simulink model "gm_dvfs_zed_simple"  (R2025b)
settings: Solver=FixedStepDiscrete  StartTime=0.0  StopTime=10.0  FixedStep=0.1  RelTol=1e-3
libraries: simulink x3
settings Model: Creator=Vimal Rency  LastModifiedBy=Vimal Rency
settings OptimizationCC: BlockReduction=off  ConditionallyExecuteInputs=off  DefaultParameterBehavior=Inlined
settings DebuggingCC: InheritedTsInSrcMsg=none
settings HardwareCC: ProdBitPerPointer=32.0  ProdBitPerSizeT=32.0  ProdBitPerPtrDiffT=32.0  ProdLargestAtomicFloat=None  ProdIntDivRoundTo=Undefined  ProdEndianess=Unspecified  ProdWordSize=32.0  ProdHWDeviceType=ASIC/FPGA->ASIC/FPGA  TargetBitPerPointer=64.0  TargetBitPerSizeT=64.0  TargetBitPerPtrDiffT=64.0  TargetLongLongMode=on  TargetIntDivRoundTo=Zero  TargetEndianess=LittleEndian  TargetWordSize=64.0  TargetHWDeviceType=Custom Processor->MATLAB Host Computer  ProdEqTarget=off

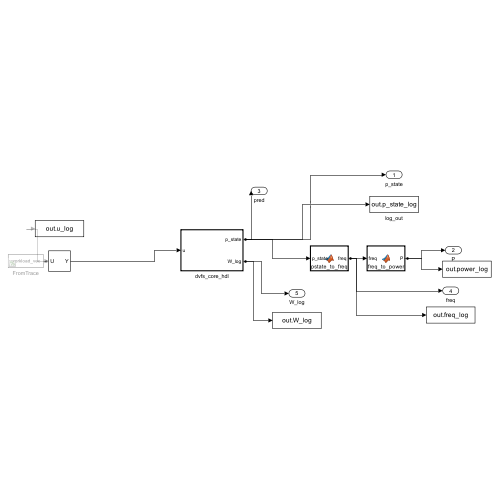
[thumbnail: Simulink's stored preview of the top-level diagram]
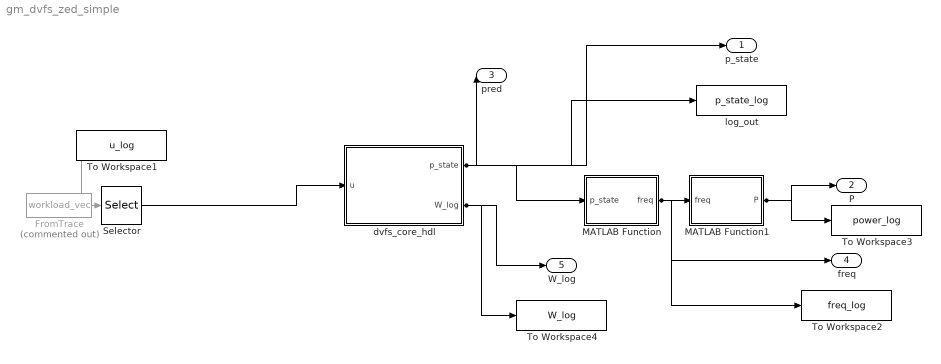
== system gm_dvfs_zed_simple ==
  FromTrace : FromWorkspace  Commented=on  VariableName=workload_vec
  MATLAB Function : MATLAB Function  TreatAsAtomicUnit=on
  MATLAB Function1 : MATLAB Function  TreatAsAtomicUnit=on
  Selector : Selector  NumberOfDimensions=2  InputPortWidth=3  IndexOptions=Select all,Index vector (dialog)  Indices=[1 3],1  OutputSizes=1,1
  To Workspace1 : ToWorkspace  VariableName=u_log  SampleTime=-1
  To Workspace2 : ToWorkspace  VariableName=freq_log  SampleTime=-1
  To Workspace3 : ToWorkspace  VariableName=power_log  SampleTime=-1
  To Workspace4 : ToWorkspace  VariableName=W_log  SampleTime=-1
  dvfs_core_hdl : Subsystem  TreatAsAtomicUnit=on
  log_out : ToWorkspace  VariableName=p_state_log  SampleTime=-1
  p_state : Outport
  P : Outport  Port=2
  pred : Outport  Port=3
  freq : Outport  Port=4
  W_log : Outport  Port=5
  wires:
  Selector/1 -> dvfs_core_hdl/1(u)
  dvfs_core_hdl/1(p_state) -> log_out/1, p_state/1, MATLAB Function/1(p_state), pred/1
  dvfs_core_hdl/2(W_log) -> W_log/1, To Workspace4/1
  MATLAB Function/1(freq) -> MATLAB Function1/1(freq), To Workspace2/1, freq/1
  MATLAB Function1/1(P) -> To Workspace3/1, P/1
  FromTrace/1 -> Selector/1, To Workspace1/1

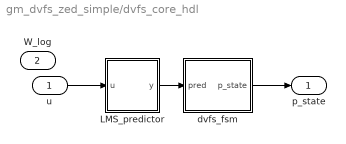
== system gm_dvfs_zed_simple/dvfs_core_hdl ==
  u : Inport  OutDataTypeStr=double  PortDimensions=1  SampleTime=0.1
  LMS_predictor : Subsystem
  dvfs_fsm : Subsystem
  p_state : Outport  SampleTime=0.1
  W_log : Outport  Port=2  SampleTime=0.1
  wires:
  u/1 -> LMS_predictor/1(u)
  LMS_predictor/1(y) -> dvfs_fsm/1(pred)
  dvfs_fsm/1(p_state) -> p_state/1

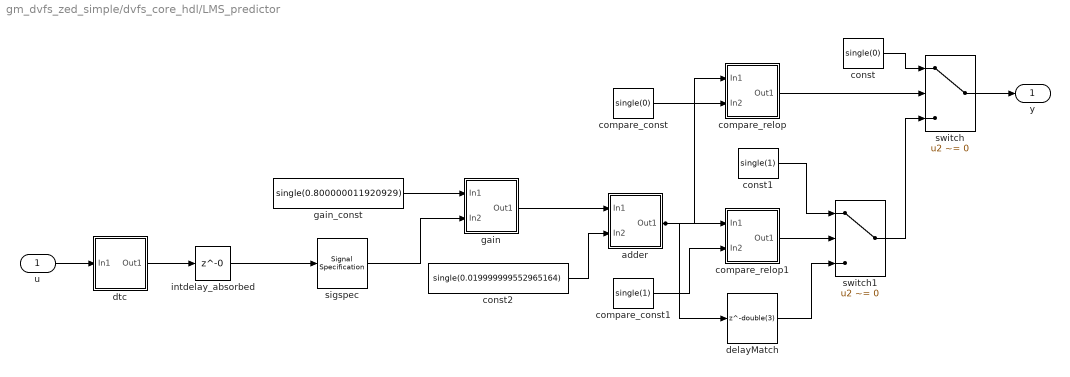
== system gm_dvfs_zed_simple/dvfs_core_hdl/LMS_predictor ==
  u : Inport  OutDataTypeStr=double  PortDimensions=1  SampleTime=0.1
  adder : Subsystem
      mask Display: disp('NFP\nadd');
  compare_const : Constant  Value=single(0)  OutDataTypeStr=single  SampleTime=0.1
  compare_const1 : Constant  Value=single(1)  OutDataTypeStr=single  SampleTime=0.1
  compare_relop : Subsystem
      mask Display: disp('NFP\nrelop');
  compare_relop1 : Subsystem
      mask Display: disp('NFP\nrelop');
  const : Constant  Value=single(0)  VectorParams1D=off  OutDataTypeStr=single  SampleTime=0.1
  const1 : Constant  Value=single(1)  VectorParams1D=off  OutDataTypeStr=single  SampleTime=0.1
  const2 : Constant  Value=single(0.019999999552965164)  VectorParams1D=off  OutDataTypeStr=single  SampleTime=0.1
  delayMatch : Delay  DelayLength=double(3)  InitialCondition=0  SampleTime=0.1
  dtc : Subsystem
      mask Display: disp('NFP\nconv');
  gain : Subsystem
      mask Display: disp('NFP\nmul');
  gain_const : Constant  Value=single(0.800000011920929)  OutDataTypeStr=single  SampleTime=0.1
  intdelay_absorbed : Delay  DelayLength=0
  sigspec : SignalSpecification  OutDataTypeStr=single  Dimensions=1
  switch : Switch  Criteria=u2 ~= 0  Threshold="fi(0,0,1,0,\"hex\",\"0\")"  OutDataTypeStr=single  SampleTime=0.1  SaturateOnIntegerOverflow=off  InputSameDT=off
  switch1 : Switch  Criteria=u2 ~= 0  Threshold="fi(0,0,1,0,\"hex\",\"0\")"  OutDataTypeStr=single  SampleTime=0.1  SaturateOnIntegerOverflow=off  InputSameDT=off
  y : Outport  SampleTime=0.1
  wires:
  u/1 -> dtc/1(In1)
  dtc/1(Out1) -> intdelay_absorbed/1
  intdelay_absorbed/1 -> sigspec/1
  gain_const/1 -> gain/1(In1)
  gain/1(Out1) -> adder/1(In1)
  sigspec/1 -> gain/2(In2)
  const2/1 -> adder/2(In2)
  compare_const/1 -> compare_relop/2(In2)
  adder/1(Out1) -> compare_relop1/1(In1), compare_relop/1(In1), delayMatch/1
  compare_const1/1 -> compare_relop1/2(In2)
  compare_relop/1(Out1) -> switch/2
  const1/1 -> switch1/1
  compare_relop1/1(Out1) -> switch1/2
  delayMatch/1 -> switch1/3
  const/1 -> switch/1
  switch1/1 -> switch/3
  switch/1 -> y/1

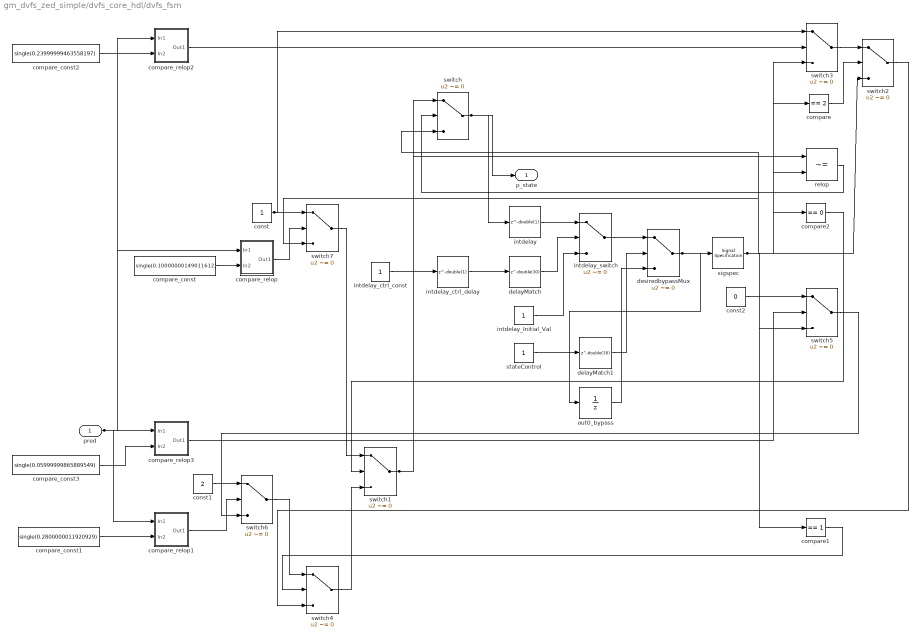
== system gm_dvfs_zed_simple/dvfs_core_hdl/dvfs_fsm ==
  pred : Inport  OutDataTypeStr=single  PortDimensions=1  SampleTime=0.1
  compare : simulink/Logic and Bit Operations/Compare To Constant  relop===  const=2  OutDataTypeStr=boolean
  compare1 : simulink/Logic and Bit Operations/Compare To Constant  relop===  const=1  OutDataTypeStr=boolean
  compare2 : simulink/Logic and Bit Operations/Compare To Constant  relop===  const=0  OutDataTypeStr=boolean
  compare_const : Constant  Value=single(0.10000000149011612)  OutDataTypeStr=single  SampleTime=0.1
  compare_const1 : Constant  Value=single(0.2800000011920929)  OutDataTypeStr=single  SampleTime=0.1
  compare_const2 : Constant  Value=single(0.23999999463558197)  OutDataTypeStr=single  SampleTime=0.1
  compare_const3 : Constant  Value=single(0.05999999865889549)  OutDataTypeStr=single  SampleTime=0.1
  compare_relop : Subsystem
      mask Display: disp('NFP\nrelop');
  compare_relop1 : Subsystem
      mask Display: disp('NFP\nrelop');
  compare_relop2 : Subsystem
      mask Display: disp('NFP\nrelop');
  compare_relop3 : Subsystem
      mask Display: disp('NFP\nrelop');
  const : Constant  VectorParams1D=off  OutDataTypeStr=uint8  SampleTime=0.1
  const1 : Constant  Value=2  VectorParams1D=off  OutDataTypeStr=uint8  SampleTime=0.1
  const2 : Constant  Value=0  VectorParams1D=off  OutDataTypeStr=uint8  SampleTime=0.1
  delayMatch : Delay  DelayLength=double(30)  InitialCondition=0  SampleTime=0.1
  delayMatch1 : Delay  DelayLength=double(30)  InitialCondition=0  SampleTime=0.1
  desiredbypassMux : Switch  Criteria=u2 ~= 0  Threshold=double(0)  OutDataTypeStr=uint8  SampleTime=0.1  SaturateOnIntegerOverflow=off  InputSameDT=off
  intdelay : Delay  DelayLength=double(1)  InitialCondition=0  SampleTime=0.1
  intdelay_Initial_Val : Constant  OutDataTypeStr=uint8  SampleTime=0.1
  intdelay_ctrl_const : Constant  OutDataTypeStr=boolean  SampleTime=0.1
  intdelay_ctrl_delay : Delay  DelayLength=double(1)  InitialCondition=0  SampleTime=0.1
  intdelay_switch : Switch  Criteria=u2 ~= 0  Threshold=double(0)  OutDataTypeStr=uint8  SampleTime=0.1  SaturateOnIntegerOverflow=off  InputSameDT=off
  out0_bypass : UnitDelay  SampleTime=0.1
  relop : RelationalOperator  Operator=~=  OutDataTypeStr=boolean  SampleTime=0.1  InputSameDT=off
  sigspec : SignalSpecification  OutDataTypeStr=uint8  Dimensions=1
  stateControl : Constant  OutDataTypeStr=boolean  SampleTime=0.1
  switch{,1..7} (8 alike) : Switch  Criteria=u2 ~= 0  Threshold="fi(0,0,1,0,\"hex\",\"0\")"  OutDataTypeStr=uint8  SampleTime=0.1  SaturateOnIntegerOverflow=off  InputSameDT=off
  p_state : Outport  SampleTime=0.1
  wires:
  const1/1 -> switch6/1
  switch7/1 -> switch1/1
  compare_const2/1 -> compare_relop2/2(In2)
  pred/1 -> compare_relop3/1(In1), compare_relop2/1(In1), compare_relop1/1(In1), compare_relop/1(In1)
  compare_const1/1 -> compare_relop1/2(In2)
  compare_const3/1 -> compare_relop3/2(In2)
  compare_relop2/1(Out1) -> switch3/2
  compare_const/1 -> compare_relop/2(In2)
  compare_relop3/1(Out1) -> switch5/2
  compare_relop1/1(Out1) -> switch6/2
  switch3/1 -> switch2/1
  const/1 -> switch7/1, switch3/1
  const2/1 -> switch5/1
  compare_relop/1(Out1) -> switch7/2
  switch6/1 -> switch4/1
  switch4/1 -> switch1/3
  switch2/1 -> switch4/3
  intdelay_ctrl_const/1 -> intdelay_ctrl_delay/1
  switch1/1 -> switch/1, relop/1
  switch/1 -> p_state/1, intdelay/1
  intdelay_ctrl_delay/1 -> delayMatch/1
  intdelay/1 -> intdelay_switch/1
  delayMatch/1 -> intdelay_switch/2
  intdelay_Initial_Val/1 -> intdelay_switch/3
  stateControl/1 -> delayMatch1/1
  intdelay_switch/1 -> desiredbypassMux/1
  delayMatch1/1 -> desiredbypassMux/2
  out0_bypass/1 -> desiredbypassMux/3
  desiredbypassMux/1 -> out0_bypass/1, sigspec/1
  sigspec/1 -> switch7/3, switch/3, switch2/3, switch5/3, switch3/3, compare1/1, compare/1, compare2/1, relop/2
  compare/1 -> switch2/2
  relop/1 -> switch/2
  compare2/1 -> switch1/2
  switch5/1 -> switch6/3
  compare1/1 -> switch4/2

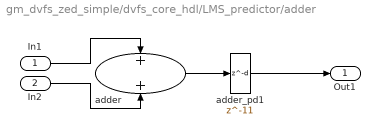
== system gm_dvfs_zed_simple/dvfs_core_hdl/LMS_predictor/adder ==
  In1 : Inport
  In2 : Inport  Port=2
  adder : Sum  OutDataTypeStr=single  SampleTime=0.1
  adder_pd1 : Delay  DelayLength=11
  Out1 : Outport
  wires:
  In1/1 -> adder/1
  In2/1 -> adder/2
  adder/1 -> adder_pd1/1
  adder_pd1/1 -> Out1/1

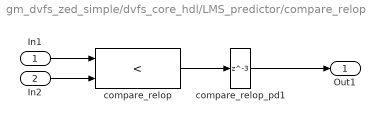
== system gm_dvfs_zed_simple/dvfs_core_hdl/LMS_predictor/compare_relop ==
  In1 : Inport
  In2 : Inport  Port=2
  compare_relop : RelationalOperator  Operator=<  OutDataTypeStr=boolean  SampleTime=0.1
  compare_relop_pd1 : Delay  DelayLength=3
  Out1 : Outport
  wires:
  In1/1 -> compare_relop/1
  In2/1 -> compare_relop/2
  compare_relop/1 -> compare_relop_pd1/1
  compare_relop_pd1/1 -> Out1/1

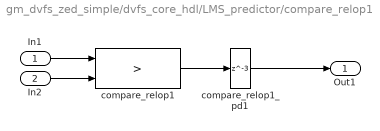
== system gm_dvfs_zed_simple/dvfs_core_hdl/LMS_predictor/compare_relop1 ==
  In1 : Inport
  In2 : Inport  Port=2
  compare_relop1 : RelationalOperator  Operator=>  OutDataTypeStr=boolean  SampleTime=0.1
  compare_relop1_pd1 : Delay  DelayLength=3
  Out1 : Outport
  wires:
  In1/1 -> compare_relop1/1
  In2/1 -> compare_relop1/2
  compare_relop1/1 -> compare_relop1_pd1/1
  compare_relop1_pd1/1 -> Out1/1

== system gm_dvfs_zed_simple/dvfs_core_hdl/LMS_predictor/dtc ==
  In1 : Inport
  dtc : DataTypeConversion  OutDataTypeStr=single  SampleTime=0.1  SaturateOnIntegerOverflow=off  RndMeth=Floor
  dtc_pd1 : Delay  DelayLength=6
  Out1 : Outport
  wires:
  In1/1 -> dtc/1
  dtc/1 -> dtc_pd1/1
  dtc_pd1/1 -> Out1/1

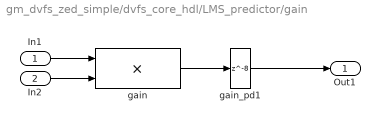
== system gm_dvfs_zed_simple/dvfs_core_hdl/LMS_predictor/gain ==
  In1 : Inport
  In2 : Inport  Port=2
  gain : Product  Inputs=**  OutDataTypeStr=single  SampleTime=0.1
  gain_pd1 : Delay  DelayLength=8
  Out1 : Outport
  wires:
  In1/1 -> gain/1
  In2/1 -> gain/2
  gain/1 -> gain_pd1/1
  gain_pd1/1 -> Out1/1

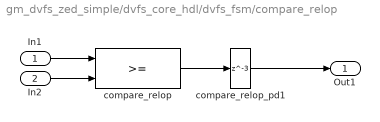
== system gm_dvfs_zed_simple/dvfs_core_hdl/dvfs_fsm/compare_relop ==
  In1 : Inport
  In2 : Inport  Port=2
  compare_relop : RelationalOperator  OutDataTypeStr=boolean  SampleTime=0.1
  compare_relop_pd1 : Delay  DelayLength=3
  Out1 : Outport
  wires:
  In1/1 -> compare_relop/1
  In2/1 -> compare_relop/2
  compare_relop/1 -> compare_relop_pd1/1
  compare_relop_pd1/1 -> Out1/1

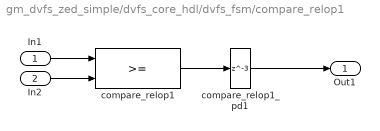
== system gm_dvfs_zed_simple/dvfs_core_hdl/dvfs_fsm/compare_relop1 ==
  In1 : Inport
  In2 : Inport  Port=2
  compare_relop1 : RelationalOperator  OutDataTypeStr=boolean  SampleTime=0.1
  compare_relop1_pd1 : Delay  DelayLength=3
  Out1 : Outport
  wires:
  In1/1 -> compare_relop1/1
  In2/1 -> compare_relop1/2
  compare_relop1/1 -> compare_relop1_pd1/1
  compare_relop1_pd1/1 -> Out1/1

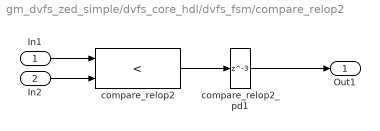
== system gm_dvfs_zed_simple/dvfs_core_hdl/dvfs_fsm/compare_relop2 ==
  In1 : Inport
  In2 : Inport  Port=2
  compare_relop2 : RelationalOperator  Operator=<  OutDataTypeStr=boolean  SampleTime=0.1
  compare_relop2_pd1 : Delay  DelayLength=3
  Out1 : Outport
  wires:
  In1/1 -> compare_relop2/1
  In2/1 -> compare_relop2/2
  compare_relop2/1 -> compare_relop2_pd1/1
  compare_relop2_pd1/1 -> Out1/1

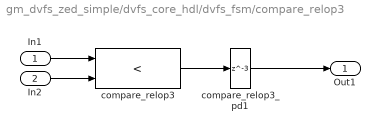
== system gm_dvfs_zed_simple/dvfs_core_hdl/dvfs_fsm/compare_relop3 ==
  In1 : Inport
  In2 : Inport  Port=2
  compare_relop3 : RelationalOperator  Operator=<  OutDataTypeStr=boolean  SampleTime=0.1
  compare_relop3_pd1 : Delay  DelayLength=3
  Out1 : Outport
  wires:
  In1/1 -> compare_relop3/1
  In2/1 -> compare_relop3/2
  compare_relop3/1 -> compare_relop3_pd1/1
  compare_relop3_pd1/1 -> Out1/1

== matlab function gm_dvfs_zed_simple/MATLAB Function1 ==
  data: freq input; P output
function P = freq_to_power(freq)

% simple model: Power ∝ frequency
P = 0.01 * freq;   % scale as you want (mW)

end

== matlab function gm_dvfs_zed_simple/MATLAB Function ==
  data: p_state input; freq output
function freq = pstate_to_freq(p_state)

switch p_state
    case 0
        freq = 100;   % MHz
    case 1
        freq = 200;
    case 2
        freq = 300;
    otherwise
        freq = 0;
end

end
